simulink model "PV_solarpannel"  (R2019b)
settings: Solver=ode45  StartTime=0.0  StopTime=10.0  RelTol=1e-3  EnableMultiTasking=on
libraries: ee_lib x243, fl_lib x39, nesl_utility x11
(part 1 of 4)
settings Model: Creator=mm  LastModifiedBy=Rishabh
settings DataIOCC: LimitDataPoints=on  SaveFormat=Array  ReturnWorkspaceOutputs=off
settings OptimizationCC: LifeSpan=inf
settings DebuggingCC: SolverPrmCheckMsg=warning  SFUnexpectedBacktrackingDiag=warning  SFNoUnconditionalDefaultTransitionDiag=warning  SFExecutionAtInitializationDiag=none  ArithmeticOperatorsInVariantConditions=warning
settings HardwareCC: ProdBitPerPointer=32  ProdBitPerSizeT=32  ProdBitPerPtrDiffT=32  ProdLargestAtomicFloat=None  ProdIntDivRoundTo=Undefined  ProdEndianess=Unspecified  ProdWordSize=32  ProdHWDeviceType=32-bit Generic
settings ModelReferenceCC: PropagateSignalLabelsOutOfModel=off
settings SFSimCC: SimUseLocalCustomCode=off  CustomCodeUndefinedFunction=UseInterfaceOnly
settings RTWCC: RTWUseLocalCustomCode=off
settings CodeAppCC: StateflowObjectComments=on
settings GRTTargetCC: TargetLangStandard=C89/C90 (ANSI)  GeneratePreprocessorConditionals=Disable all
settings ConfigComp: CovMetricSettings=dw  CovHtmlReporting=on  CovSaveCumulativeToWorkspaceVar=on  CovSaveSingleToWorkspaceVar=on  CovExternalEMLEnable=off  CovSFcnEnable=off
settings SimscapeCC: SimscapeNormalizeSystem=off

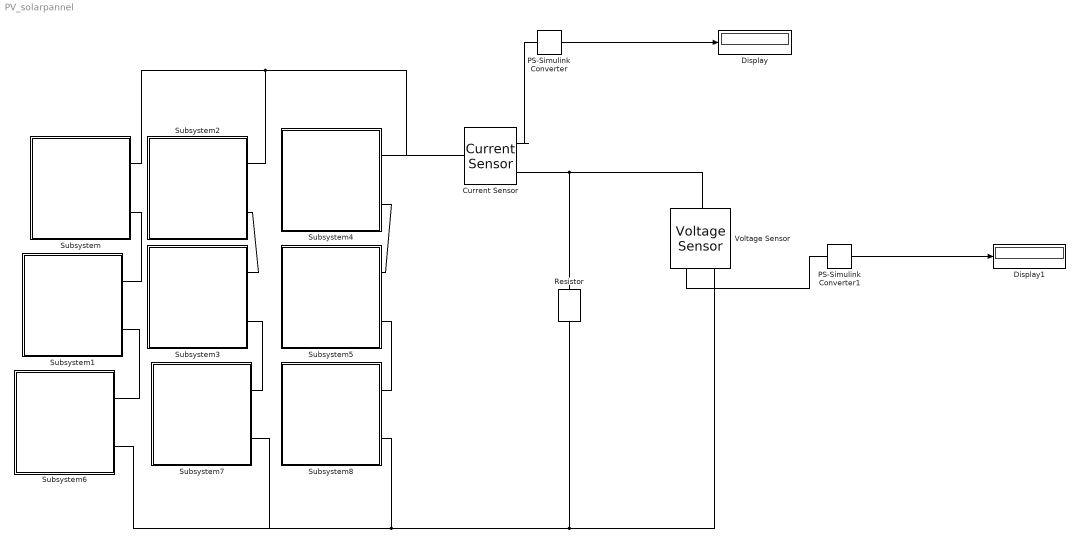
== system PV_solarpannel ==
  Current Sensor : fl_lib/Electrical/Electrical Sensors/Current Sensor
  Display : Display
  Display1 : Display
  PS-Simulink Converter : nesl_utility/PS-Simulink Converter  PhysicalDomain=network_engine_domain  SubClassName=ps_output  LeftPortType=input  RightPortType=output  PseudoPeriodic=off  Frequencies=[]  Unit=1  AffineConversion=off
  PS-Simulink Converter1 : nesl_utility/PS-Simulink Converter  PhysicalDomain=network_engine_domain  SubClassName=ps_output  LeftPortType=input  RightPortType=output  PseudoPeriodic=off  Frequencies=[]  Unit=1  AffineConversion=off
  Resistor : fl_lib/Electrical/Electrical Elements/Resistor  R=1 Ohm  i_specify=off  i_priority=High  i=0 A  i_nominal_specify=off  i_nominal_unit=A  i_nominal_value=1  v_specify=off  v_priority=High  v=0 V  v_nominal_specify=off  v_nominal_unit=V  v_nominal_value=1
  Subsystem : Subsystem
  Subsystem1 : Subsystem
  Subsystem2 : Subsystem
  Subsystem3 : Subsystem
  Subsystem4 : Subsystem
  Subsystem5 : Subsystem
  Subsystem6 : Subsystem
  Subsystem7 : Subsystem
  Subsystem8 : Subsystem
  Voltage Sensor : fl_lib/Electrical/Electrical Sensors/Voltage Sensor
  wires:
  PS-Simulink Converter/1 -> Display/1
  PS-Simulink Converter1/1 -> Display1/1
  connections:
  Current Sensor/RConn2 -- Voltage Sensor/LConn1 -- Resistor/LConn1
  Current Sensor/RConn1 -- PS-Simulink Converter/LConn1
  Voltage Sensor/RConn1 -- PS-Simulink Converter1/LConn1
  Resistor/RConn1 -- Subsystem7/RConn2 -- Subsystem6/RConn2 -- Subsystem8/RConn2 -- Voltage Sensor/RConn2
  Subsystem1/RConn1 -- Subsystem/RConn2
  Subsystem3/RConn1 -- Subsystem2/RConn2
  Subsystem3/RConn2 -- Subsystem7/RConn1
  Subsystem1/RConn2 -- Subsystem6/RConn1
  Subsystem5/RConn2 -- Subsystem8/RConn1
  Subsystem4/RConn2 -- Subsystem5/RConn1
  Subsystem/RConn1 -- Subsystem4/RConn1 -- Current Sensor/LConn1 -- Subsystem2/RConn1

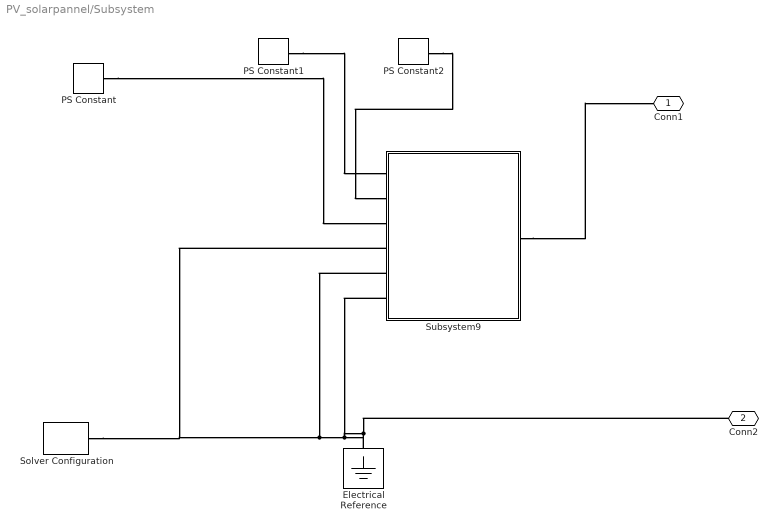
== system PV_solarpannel/Subsystem ==
  Electrical Reference : fl_lib/Electrical/Electrical Elements/Electrical Reference
  PS Constant : fl_lib/Physical Signals/Sources/PS Constant  constant=1000
  PS Constant1 : fl_lib/Physical Signals/Sources/PS Constant  constant=1000
  PS Constant2 : fl_lib/Physical Signals/Sources/PS Constant  constant=1000
  Solver Configuration : nesl_utility/Solver Configuration  PhysicalDomain=network_engine_domain  SubClassName=solver  LeftPortType=input  RightPortType=generic  Tones=[]  Harmonics=[]  SimulateNoise=off  Profile=off  UseLocalSampling=off  EnableSwitchedLinearOptims=on  FrequencyDomain=off  UseCCode=off  RelTol=0.001  AbsTol=1e-06  MinStep=1e-09  ToWorkspace=off  RevertToSquareIcSolve=off  NumHomotopyIterations=100  PhasorMode=off  PhasorModeNumHarmonics=1  DoDC=off  ResidualTolerance=1e-09  UseLocalSolver=off  LocalSolverChoice=NE_BACKWARD_EULER_ADVANCER  LocalSolverSampleTime=0.001  DoFixedCost=off  MaxNonlinIter=3  MaxModeIter=2  LinearAlgebra=Sparse  EquationFormulation=NE_TIME_EF  DelaysMemoryBudget=1024  AutomaticFiltering=on  FilteringTimeConstant=0.001  PartitionStorageMethod=AS_NEEDED  PartitionMemoryBudget=1024  PartitionMethod=FAST
  Subsystem9 : Subsystem
  Conn1 : PMIOPort  Side=Right
  Conn2 : PMIOPort  Port=2  Side=Right
  connections:
  Electrical Reference/LConn1 -- Subsystem9/LConn6 -- Subsystem9/LConn5 -- Subsystem9/LConn4 -- Solver Configuration/RConn1 -- Conn2/RConn1
  PS Constant1/RConn1 -- Subsystem9/LConn1
  PS Constant/RConn1 -- Subsystem9/LConn3
  PS Constant2/RConn1 -- Subsystem9/LConn2
  Subsystem9/RConn1 -- Conn1/RConn1

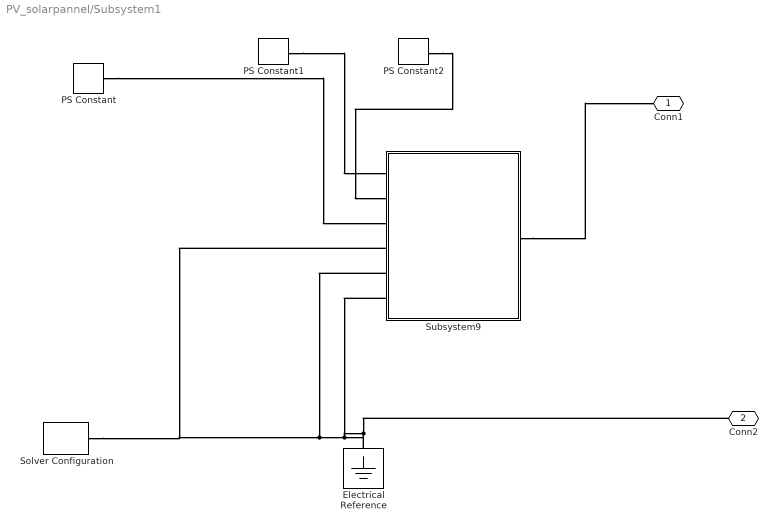
== system PV_solarpannel/Subsystem1 ==
  Electrical Reference : fl_lib/Electrical/Electrical Elements/Electrical Reference
  PS Constant : fl_lib/Physical Signals/Sources/PS Constant  constant=1000
  PS Constant1 : fl_lib/Physical Signals/Sources/PS Constant  constant=1000
  PS Constant2 : fl_lib/Physical Signals/Sources/PS Constant  constant=1000
  Solver Configuration : nesl_utility/Solver Configuration  PhysicalDomain=network_engine_domain  SubClassName=solver  LeftPortType=input  RightPortType=generic  Tones=[]  Harmonics=[]  SimulateNoise=off  Profile=off  UseLocalSampling=off  EnableSwitchedLinearOptims=on  FrequencyDomain=off  UseCCode=off  RelTol=0.001  AbsTol=1e-06  MinStep=1e-09  ToWorkspace=off  RevertToSquareIcSolve=off  NumHomotopyIterations=100  PhasorMode=off  PhasorModeNumHarmonics=1  DoDC=off  ResidualTolerance=1e-09  UseLocalSolver=off  LocalSolverChoice=NE_BACKWARD_EULER_ADVANCER  LocalSolverSampleTime=0.001  DoFixedCost=off  MaxNonlinIter=3  MaxModeIter=2  LinearAlgebra=Sparse  EquationFormulation=NE_TIME_EF  DelaysMemoryBudget=1024  AutomaticFiltering=on  FilteringTimeConstant=0.001  PartitionStorageMethod=AS_NEEDED  PartitionMemoryBudget=1024  PartitionMethod=FAST
  Subsystem9 : Subsystem
  Conn1 : PMIOPort  Side=Right
  Conn2 : PMIOPort  Port=2  Side=Right
  connections:
  Electrical Reference/LConn1 -- Subsystem9/LConn6 -- Subsystem9/LConn5 -- Subsystem9/LConn4 -- Solver Configuration/RConn1 -- Conn2/RConn1
  PS Constant1/RConn1 -- Subsystem9/LConn1
  PS Constant/RConn1 -- Subsystem9/LConn3
  PS Constant2/RConn1 -- Subsystem9/LConn2
  Subsystem9/RConn1 -- Conn1/RConn1

== system PV_solarpannel/Subsystem2 ==
  Electrical Reference : fl_lib/Electrical/Electrical Elements/Electrical Reference
  PS Constant : fl_lib/Physical Signals/Sources/PS Constant  constant=1000
  PS Constant1 : fl_lib/Physical Signals/Sources/PS Constant  constant=1000
  PS Constant2 : fl_lib/Physical Signals/Sources/PS Constant  constant=1000
  Solver Configuration : nesl_utility/Solver Configuration  PhysicalDomain=network_engine_domain  SubClassName=solver  LeftPortType=input  RightPortType=generic  Tones=[]  Harmonics=[]  SimulateNoise=off  Profile=off  UseLocalSampling=off  EnableSwitchedLinearOptims=on  FrequencyDomain=off  UseCCode=off  RelTol=0.001  AbsTol=1e-06  MinStep=1e-09  ToWorkspace=off  RevertToSquareIcSolve=off  NumHomotopyIterations=100  PhasorMode=off  PhasorModeNumHarmonics=1  DoDC=off  ResidualTolerance=1e-09  UseLocalSolver=off  LocalSolverChoice=NE_BACKWARD_EULER_ADVANCER  LocalSolverSampleTime=0.001  DoFixedCost=off  MaxNonlinIter=3  MaxModeIter=2  LinearAlgebra=Sparse  EquationFormulation=NE_TIME_EF  DelaysMemoryBudget=1024  AutomaticFiltering=on  FilteringTimeConstant=0.001  PartitionStorageMethod=AS_NEEDED  PartitionMemoryBudget=1024  PartitionMethod=FAST
  Subsystem9 : Subsystem
  Conn1 : PMIOPort  Side=Right
  Conn2 : PMIOPort  Port=2  Side=Right
  connections:
  Electrical Reference/LConn1 -- Subsystem9/LConn6 -- Subsystem9/LConn5 -- Subsystem9/LConn4 -- Solver Configuration/RConn1 -- Conn2/RConn1
  PS Constant1/RConn1 -- Subsystem9/LConn1
  PS Constant/RConn1 -- Subsystem9/LConn3
  PS Constant2/RConn1 -- Subsystem9/LConn2
  Subsystem9/RConn1 -- Conn1/RConn1

== system PV_solarpannel/Subsystem3 ==
  Electrical Reference : fl_lib/Electrical/Electrical Elements/Electrical Reference
  PS Constant : fl_lib/Physical Signals/Sources/PS Constant  constant=1000
  PS Constant1 : fl_lib/Physical Signals/Sources/PS Constant  constant=1000
  PS Constant2 : fl_lib/Physical Signals/Sources/PS Constant  constant=1000
  Solver Configuration : nesl_utility/Solver Configuration  PhysicalDomain=network_engine_domain  SubClassName=solver  LeftPortType=input  RightPortType=generic  Tones=[]  Harmonics=[]  SimulateNoise=off  Profile=off  UseLocalSampling=off  EnableSwitchedLinearOptims=on  FrequencyDomain=off  UseCCode=off  RelTol=0.001  AbsTol=1e-06  MinStep=1e-09  ToWorkspace=off  RevertToSquareIcSolve=off  NumHomotopyIterations=100  PhasorMode=off  PhasorModeNumHarmonics=1  DoDC=off  ResidualTolerance=1e-09  UseLocalSolver=off  LocalSolverChoice=NE_BACKWARD_EULER_ADVANCER  LocalSolverSampleTime=0.001  DoFixedCost=off  MaxNonlinIter=3  MaxModeIter=2  LinearAlgebra=Sparse  EquationFormulation=NE_TIME_EF  DelaysMemoryBudget=1024  AutomaticFiltering=on  FilteringTimeConstant=0.001  PartitionStorageMethod=AS_NEEDED  PartitionMemoryBudget=1024  PartitionMethod=FAST
  Subsystem9 : Subsystem
  Conn1 : PMIOPort  Side=Right
  Conn2 : PMIOPort  Port=2  Side=Right
  connections:
  Electrical Reference/LConn1 -- Subsystem9/LConn6 -- Subsystem9/LConn5 -- Subsystem9/LConn4 -- Solver Configuration/RConn1 -- Conn2/RConn1
  PS Constant1/RConn1 -- Subsystem9/LConn1
  PS Constant/RConn1 -- Subsystem9/LConn3
  PS Constant2/RConn1 -- Subsystem9/LConn2
  Subsystem9/RConn1 -- Conn1/RConn1

== system PV_solarpannel/Subsystem4 ==
  Electrical Reference : fl_lib/Electrical/Electrical Elements/Electrical Reference
  PS Constant : fl_lib/Physical Signals/Sources/PS Constant  constant=1000
  PS Constant1 : fl_lib/Physical Signals/Sources/PS Constant  constant=1000
  PS Constant2 : fl_lib/Physical Signals/Sources/PS Constant  constant=1000
  Solver Configuration : nesl_utility/Solver Configuration  PhysicalDomain=network_engine_domain  SubClassName=solver  LeftPortType=input  RightPortType=generic  Tones=[]  Harmonics=[]  SimulateNoise=off  Profile=off  UseLocalSampling=off  EnableSwitchedLinearOptims=on  FrequencyDomain=off  UseCCode=off  RelTol=0.001  AbsTol=1e-06  MinStep=1e-09  ToWorkspace=off  RevertToSquareIcSolve=off  NumHomotopyIterations=100  PhasorMode=off  PhasorModeNumHarmonics=1  DoDC=off  ResidualTolerance=1e-09  UseLocalSolver=off  LocalSolverChoice=NE_BACKWARD_EULER_ADVANCER  LocalSolverSampleTime=0.001  DoFixedCost=off  MaxNonlinIter=3  MaxModeIter=2  LinearAlgebra=Sparse  EquationFormulation=NE_TIME_EF  DelaysMemoryBudget=1024  AutomaticFiltering=on  FilteringTimeConstant=0.001  PartitionStorageMethod=AS_NEEDED  PartitionMemoryBudget=1024  PartitionMethod=FAST
  Subsystem9 : Subsystem
  Conn1 : PMIOPort  Side=Right
  Conn2 : PMIOPort  Port=2  Side=Right
  connections:
  Electrical Reference/LConn1 -- Subsystem9/LConn6 -- Subsystem9/LConn5 -- Subsystem9/LConn4 -- Solver Configuration/RConn1 -- Conn2/RConn1
  PS Constant1/RConn1 -- Subsystem9/LConn1
  PS Constant/RConn1 -- Subsystem9/LConn3
  PS Constant2/RConn1 -- Subsystem9/LConn2
  Subsystem9/RConn1 -- Conn1/RConn1

== system PV_solarpannel/Subsystem5 ==
  Electrical Reference : fl_lib/Electrical/Electrical Elements/Electrical Reference
  PS Constant : fl_lib/Physical Signals/Sources/PS Constant  constant=1000
  PS Constant1 : fl_lib/Physical Signals/Sources/PS Constant  constant=1000
  PS Constant2 : fl_lib/Physical Signals/Sources/PS Constant  constant=1000
  Solver Configuration : nesl_utility/Solver Configuration  PhysicalDomain=network_engine_domain  SubClassName=solver  LeftPortType=input  RightPortType=generic  Tones=[]  Harmonics=[]  SimulateNoise=off  Profile=off  UseLocalSampling=off  EnableSwitchedLinearOptims=on  FrequencyDomain=off  UseCCode=off  RelTol=0.001  AbsTol=1e-06  MinStep=1e-09  ToWorkspace=off  RevertToSquareIcSolve=off  NumHomotopyIterations=100  PhasorMode=off  PhasorModeNumHarmonics=1  DoDC=off  ResidualTolerance=1e-09  UseLocalSolver=off  LocalSolverChoice=NE_BACKWARD_EULER_ADVANCER  LocalSolverSampleTime=0.001  DoFixedCost=off  MaxNonlinIter=3  MaxModeIter=2  LinearAlgebra=Sparse  EquationFormulation=NE_TIME_EF  DelaysMemoryBudget=1024  AutomaticFiltering=on  FilteringTimeConstant=0.001  PartitionStorageMethod=AS_NEEDED  PartitionMemoryBudget=1024  PartitionMethod=FAST
  Subsystem9 : Subsystem
  Conn1 : PMIOPort  Side=Right
  Conn2 : PMIOPort  Port=2  Side=Right
  connections:
  Electrical Reference/LConn1 -- Subsystem9/LConn6 -- Subsystem9/LConn5 -- Subsystem9/LConn4 -- Solver Configuration/RConn1 -- Conn2/RConn1
  PS Constant1/RConn1 -- Subsystem9/LConn1
  PS Constant/RConn1 -- Subsystem9/LConn3
  PS Constant2/RConn1 -- Subsystem9/LConn2
  Subsystem9/RConn1 -- Conn1/RConn1

== system PV_solarpannel/Subsystem6 ==
  Electrical Reference : fl_lib/Electrical/Electrical Elements/Electrical Reference
  PS Constant : fl_lib/Physical Signals/Sources/PS Constant  constant=1000
  PS Constant1 : fl_lib/Physical Signals/Sources/PS Constant  constant=1000
  PS Constant2 : fl_lib/Physical Signals/Sources/PS Constant  constant=1000
  Solver Configuration : nesl_utility/Solver Configuration  PhysicalDomain=network_engine_domain  SubClassName=solver  LeftPortType=input  RightPortType=generic  Tones=[]  Harmonics=[]  SimulateNoise=off  Profile=off  UseLocalSampling=off  EnableSwitchedLinearOptims=on  FrequencyDomain=off  UseCCode=off  RelTol=0.001  AbsTol=1e-06  MinStep=1e-09  ToWorkspace=off  RevertToSquareIcSolve=off  NumHomotopyIterations=100  PhasorMode=off  PhasorModeNumHarmonics=1  DoDC=off  ResidualTolerance=1e-09  UseLocalSolver=off  LocalSolverChoice=NE_BACKWARD_EULER_ADVANCER  LocalSolverSampleTime=0.001  DoFixedCost=off  MaxNonlinIter=3  MaxModeIter=2  LinearAlgebra=Sparse  EquationFormulation=NE_TIME_EF  DelaysMemoryBudget=1024  AutomaticFiltering=on  FilteringTimeConstant=0.001  PartitionStorageMethod=AS_NEEDED  PartitionMemoryBudget=1024  PartitionMethod=FAST
  Subsystem9 : Subsystem
  Conn1 : PMIOPort  Side=Right
  Conn2 : PMIOPort  Port=2  Side=Right
  connections:
  Electrical Reference/LConn1 -- Subsystem9/LConn6 -- Subsystem9/LConn5 -- Subsystem9/LConn4 -- Solver Configuration/RConn1 -- Conn2/RConn1
  PS Constant1/RConn1 -- Subsystem9/LConn1
  PS Constant/RConn1 -- Subsystem9/LConn3
  PS Constant2/RConn1 -- Subsystem9/LConn2
  Subsystem9/RConn1 -- Conn1/RConn1

== system PV_solarpannel/Subsystem7 ==
  Electrical Reference : fl_lib/Electrical/Electrical Elements/Electrical Reference
  PS Constant : fl_lib/Physical Signals/Sources/PS Constant  constant=1000
  PS Constant1 : fl_lib/Physical Signals/Sources/PS Constant  constant=1000
  PS Constant2 : fl_lib/Physical Signals/Sources/PS Constant  constant=1000
  Solver Configuration : nesl_utility/Solver Configuration  PhysicalDomain=network_engine_domain  SubClassName=solver  LeftPortType=input  RightPortType=generic  Tones=[]  Harmonics=[]  SimulateNoise=off  Profile=off  UseLocalSampling=off  EnableSwitchedLinearOptims=on  FrequencyDomain=off  UseCCode=off  RelTol=0.001  AbsTol=1e-06  MinStep=1e-09  ToWorkspace=off  RevertToSquareIcSolve=off  NumHomotopyIterations=100  PhasorMode=off  PhasorModeNumHarmonics=1  DoDC=off  ResidualTolerance=1e-09  UseLocalSolver=off  LocalSolverChoice=NE_BACKWARD_EULER_ADVANCER  LocalSolverSampleTime=0.001  DoFixedCost=off  MaxNonlinIter=3  MaxModeIter=2  LinearAlgebra=Sparse  EquationFormulation=NE_TIME_EF  DelaysMemoryBudget=1024  AutomaticFiltering=on  FilteringTimeConstant=0.001  PartitionStorageMethod=AS_NEEDED  PartitionMemoryBudget=1024  PartitionMethod=FAST
  Subsystem9 : Subsystem
  Conn1 : PMIOPort  Side=Right
  Conn2 : PMIOPort  Port=2  Side=Right
  connections:
  Electrical Reference/LConn1 -- Subsystem9/LConn6 -- Subsystem9/LConn5 -- Subsystem9/LConn4 -- Solver Configuration/RConn1 -- Conn2/RConn1
  PS Constant1/RConn1 -- Subsystem9/LConn1
  PS Constant/RConn1 -- Subsystem9/LConn3
  PS Constant2/RConn1 -- Subsystem9/LConn2
  Subsystem9/RConn1 -- Conn1/RConn1

== system PV_solarpannel/Subsystem8 ==
  Electrical Reference : fl_lib/Electrical/Electrical Elements/Electrical Reference
  PS Constant : fl_lib/Physical Signals/Sources/PS Constant  constant=1000
  PS Constant1 : fl_lib/Physical Signals/Sources/PS Constant  constant=1000
  PS Constant2 : fl_lib/Physical Signals/Sources/PS Constant  constant=1000
  Solver Configuration : nesl_utility/Solver Configuration  PhysicalDomain=network_engine_domain  SubClassName=solver  LeftPortType=input  RightPortType=generic  Tones=[]  Harmonics=[]  SimulateNoise=off  Profile=off  UseLocalSampling=off  EnableSwitchedLinearOptims=on  FrequencyDomain=off  UseCCode=off  RelTol=0.001  AbsTol=1e-06  MinStep=1e-09  ToWorkspace=off  RevertToSquareIcSolve=off  NumHomotopyIterations=100  PhasorMode=off  PhasorModeNumHarmonics=1  DoDC=off  ResidualTolerance=1e-09  UseLocalSolver=off  LocalSolverChoice=NE_BACKWARD_EULER_ADVANCER  LocalSolverSampleTime=0.001  DoFixedCost=off  MaxNonlinIter=3  MaxModeIter=2  LinearAlgebra=Sparse  EquationFormulation=NE_TIME_EF  DelaysMemoryBudget=1024  AutomaticFiltering=on  FilteringTimeConstant=0.001  PartitionStorageMethod=AS_NEEDED  PartitionMemoryBudget=1024  PartitionMethod=FAST
  Subsystem9 : Subsystem
  Conn1 : PMIOPort  Side=Right
  Conn2 : PMIOPort  Port=2  Side=Right
  connections:
  Electrical Reference/LConn1 -- Subsystem9/LConn6 -- Subsystem9/LConn5 -- Subsystem9/LConn4 -- Solver Configuration/RConn1 -- Conn2/RConn1
  PS Constant1/RConn1 -- Subsystem9/LConn1
  PS Constant/RConn1 -- Subsystem9/LConn3
  PS Constant2/RConn1 -- Subsystem9/LConn2
  Subsystem9/RConn1 -- Conn1/RConn1

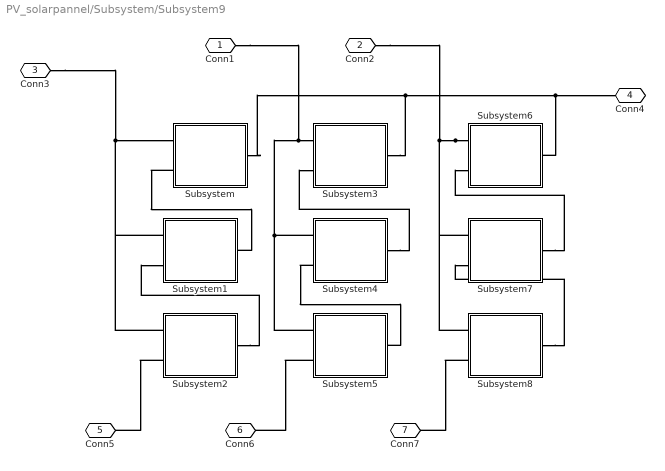
== system PV_solarpannel/Subsystem/Subsystem9 ==
  Subsystem : Subsystem
  Subsystem1 : Subsystem
  Subsystem2 : Subsystem
  Subsystem3 : Subsystem
  Subsystem4 : Subsystem
  Subsystem5 : Subsystem
  Subsystem6 : Subsystem
  Subsystem7 : Subsystem
  Subsystem8 : Subsystem
  Conn1 : PMIOPort  Side=Left
  Conn2 : PMIOPort  Port=2  Side=Left
  Conn3 : PMIOPort  Port=3  Side=Left
  Conn4 : PMIOPort  Port=4  Side=Right
  Conn5 : PMIOPort  Port=5  Side=Left
  Conn6 : PMIOPort  Port=6  Side=Left
  Conn7 : PMIOPort  Port=7  Side=Left
  connections:
  Subsystem3/RConn1 -- Subsystem/RConn1 -- Conn4/RConn1 -- Subsystem6/RConn1
  Subsystem6/LConn1 -- Conn2/RConn1 -- Subsystem8/LConn1 -- Subsystem7/LConn1
  Subsystem8/RConn1 -- Subsystem7/LConn2
  Subsystem4/LConn1 -- Conn1/RConn1 -- Subsystem3/LConn1 -- Subsystem5/LConn1
  Subsystem2/LConn2 -- Conn5/RConn1
  Subsystem/LConn2 -- Subsystem1/RConn1
  Subsystem7/RConn1 -- Subsystem6/LConn2
  Subsystem2/LConn1 -- Subsystem1/LConn1 -- Conn3/RConn1 -- Subsystem/LConn1
  Subsystem2/RConn1 -- Subsystem1/LConn2
  Subsystem4/RConn1 -- Subsystem3/LConn2
  Subsystem4/LConn2 -- Subsystem5/RConn1
  Subsystem8/LConn2 -- Conn7/RConn1
  Subsystem5/LConn2 -- Conn6/RConn1

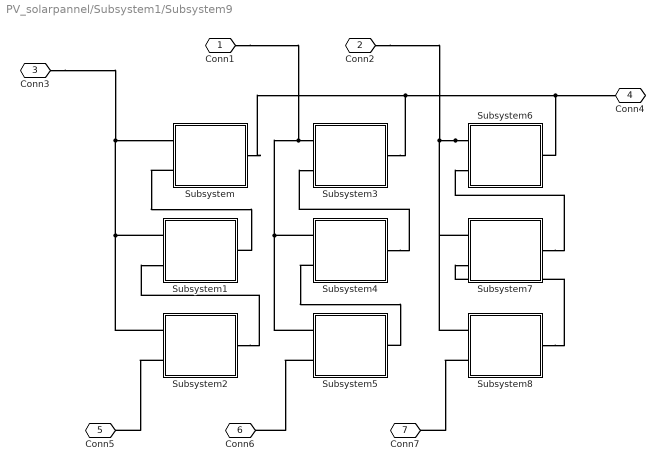
== system PV_solarpannel/Subsystem1/Subsystem9 ==
  Subsystem : Subsystem
  Subsystem1 : Subsystem
  Subsystem2 : Subsystem
  Subsystem3 : Subsystem
  Subsystem4 : Subsystem
  Subsystem5 : Subsystem
  Subsystem6 : Subsystem
  Subsystem7 : Subsystem
  Subsystem8 : Subsystem
  Conn1 : PMIOPort  Side=Left
  Conn2 : PMIOPort  Port=2  Side=Left
  Conn3 : PMIOPort  Port=3  Side=Left
  Conn4 : PMIOPort  Port=4  Side=Right
  Conn5 : PMIOPort  Port=5  Side=Left
  Conn6 : PMIOPort  Port=6  Side=Left
  Conn7 : PMIOPort  Port=7  Side=Left
  connections:
  Subsystem3/RConn1 -- Subsystem/RConn1 -- Conn4/RConn1 -- Subsystem6/RConn1
  Subsystem6/LConn1 -- Conn2/RConn1 -- Subsystem8/LConn1 -- Subsystem7/LConn1
  Subsystem8/RConn1 -- Subsystem7/LConn2
  Subsystem4/LConn1 -- Conn1/RConn1 -- Subsystem3/LConn1 -- Subsystem5/LConn1
  Subsystem2/LConn2 -- Conn5/RConn1
  Subsystem/LConn2 -- Subsystem1/RConn1
  Subsystem7/RConn1 -- Subsystem6/LConn2
  Subsystem2/LConn1 -- Subsystem1/LConn1 -- Conn3/RConn1 -- Subsystem/LConn1
  Subsystem2/RConn1 -- Subsystem1/LConn2
  Subsystem4/RConn1 -- Subsystem3/LConn2
  Subsystem4/LConn2 -- Subsystem5/RConn1
  Subsystem8/LConn2 -- Conn7/RConn1
  Subsystem5/LConn2 -- Conn6/RConn1

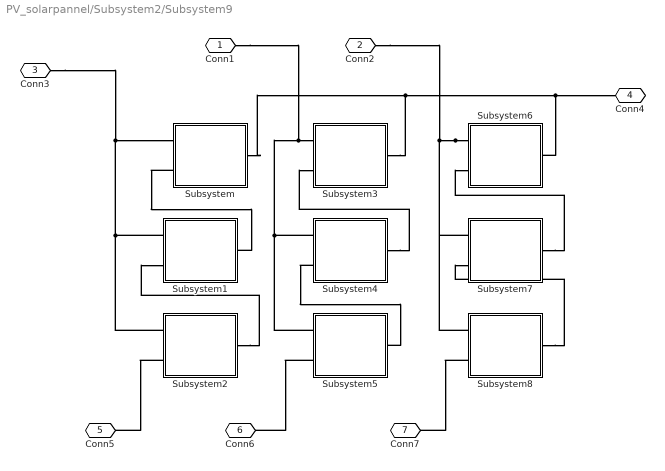
== system PV_solarpannel/Subsystem2/Subsystem9 ==
  Subsystem : Subsystem
  Subsystem1 : Subsystem
  Subsystem2 : Subsystem
  Subsystem3 : Subsystem
  Subsystem4 : Subsystem
  Subsystem5 : Subsystem
  Subsystem6 : Subsystem
  Subsystem7 : Subsystem
  Subsystem8 : Subsystem
  Conn1 : PMIOPort  Side=Left
  Conn2 : PMIOPort  Port=2  Side=Left
  Conn3 : PMIOPort  Port=3  Side=Left
  Conn4 : PMIOPort  Port=4  Side=Right
  Conn5 : PMIOPort  Port=5  Side=Left
  Conn6 : PMIOPort  Port=6  Side=Left
  Conn7 : PMIOPort  Port=7  Side=Left
  connections:
  Subsystem3/RConn1 -- Subsystem/RConn1 -- Conn4/RConn1 -- Subsystem6/RConn1
  Subsystem6/LConn1 -- Conn2/RConn1 -- Subsystem8/LConn1 -- Subsystem7/LConn1
  Subsystem8/RConn1 -- Subsystem7/LConn2
  Subsystem4/LConn1 -- Conn1/RConn1 -- Subsystem3/LConn1 -- Subsystem5/LConn1
  Subsystem2/LConn2 -- Conn5/RConn1
  Subsystem/LConn2 -- Subsystem1/RConn1
  Subsystem7/RConn1 -- Subsystem6/LConn2
  Subsystem2/LConn1 -- Subsystem1/LConn1 -- Conn3/RConn1 -- Subsystem/LConn1
  Subsystem2/RConn1 -- Subsystem1/LConn2
  Subsystem4/RConn1 -- Subsystem3/LConn2
  Subsystem4/LConn2 -- Subsystem5/RConn1
  Subsystem8/LConn2 -- Conn7/RConn1
  Subsystem5/LConn2 -- Conn6/RConn1

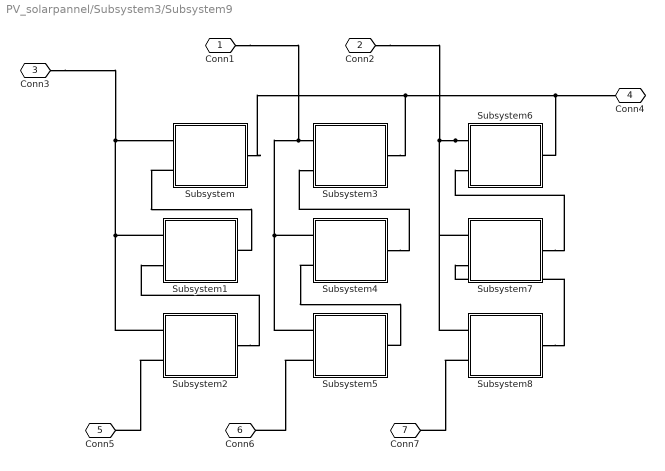
== system PV_solarpannel/Subsystem3/Subsystem9 ==
  Subsystem : Subsystem
  Subsystem1 : Subsystem
  Subsystem2 : Subsystem
  Subsystem3 : Subsystem
  Subsystem4 : Subsystem
  Subsystem5 : Subsystem
  Subsystem6 : Subsystem
  Subsystem7 : Subsystem
  Subsystem8 : Subsystem
  Conn1 : PMIOPort  Side=Left
  Conn2 : PMIOPort  Port=2  Side=Left
  Conn3 : PMIOPort  Port=3  Side=Left
  Conn4 : PMIOPort  Port=4  Side=Right
  Conn5 : PMIOPort  Port=5  Side=Left
  Conn6 : PMIOPort  Port=6  Side=Left
  Conn7 : PMIOPort  Port=7  Side=Left
  connections:
  Subsystem3/RConn1 -- Subsystem/RConn1 -- Conn4/RConn1 -- Subsystem6/RConn1
  Subsystem6/LConn1 -- Conn2/RConn1 -- Subsystem8/LConn1 -- Subsystem7/LConn1
  Subsystem8/RConn1 -- Subsystem7/LConn2
  Subsystem4/LConn1 -- Conn1/RConn1 -- Subsystem3/LConn1 -- Subsystem5/LConn1
  Subsystem2/LConn2 -- Conn5/RConn1
  Subsystem/LConn2 -- Subsystem1/RConn1
  Subsystem7/RConn1 -- Subsystem6/LConn2
  Subsystem2/LConn1 -- Subsystem1/LConn1 -- Conn3/RConn1 -- Subsystem/LConn1
  Subsystem2/RConn1 -- Subsystem1/LConn2
  Subsystem4/RConn1 -- Subsystem3/LConn2
  Subsystem4/LConn2 -- Subsystem5/RConn1
  Subsystem8/LConn2 -- Conn7/RConn1
  Subsystem5/LConn2 -- Conn6/RConn1

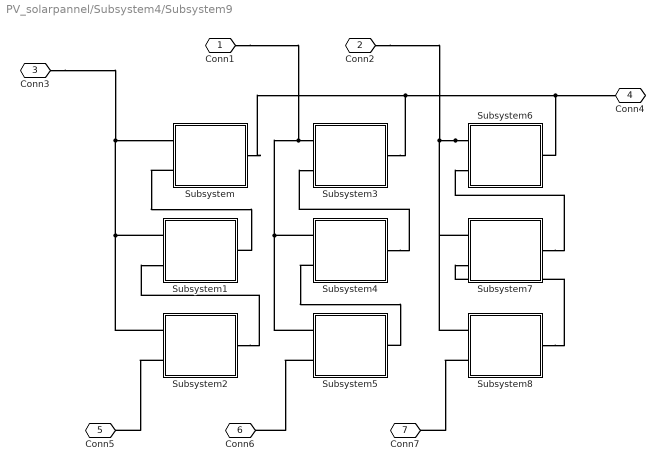
== system PV_solarpannel/Subsystem4/Subsystem9 ==
  Subsystem : Subsystem
  Subsystem1 : Subsystem
  Subsystem2 : Subsystem
  Subsystem3 : Subsystem
  Subsystem4 : Subsystem
  Subsystem5 : Subsystem
  Subsystem6 : Subsystem
  Subsystem7 : Subsystem
  Subsystem8 : Subsystem
  Conn1 : PMIOPort  Side=Left
  Conn2 : PMIOPort  Port=2  Side=Left
  Conn3 : PMIOPort  Port=3  Side=Left
  Conn4 : PMIOPort  Port=4  Side=Right
  Conn5 : PMIOPort  Port=5  Side=Left
  Conn6 : PMIOPort  Port=6  Side=Left
  Conn7 : PMIOPort  Port=7  Side=Left
  connections:
  Subsystem3/RConn1 -- Subsystem/RConn1 -- Conn4/RConn1 -- Subsystem6/RConn1
  Subsystem6/LConn1 -- Conn2/RConn1 -- Subsystem8/LConn1 -- Subsystem7/LConn1
  Subsystem8/RConn1 -- Subsystem7/LConn2
  Subsystem4/LConn1 -- Conn1/RConn1 -- Subsystem3/LConn1 -- Subsystem5/LConn1
  Subsystem2/LConn2 -- Conn5/RConn1
  Subsystem/LConn2 -- Subsystem1/RConn1
  Subsystem7/RConn1 -- Subsystem6/LConn2
  Subsystem2/LConn1 -- Subsystem1/LConn1 -- Conn3/RConn1 -- Subsystem/LConn1
  Subsystem2/RConn1 -- Subsystem1/LConn2
  Subsystem4/RConn1 -- Subsystem3/LConn2
  Subsystem4/LConn2 -- Subsystem5/RConn1
  Subsystem8/LConn2 -- Conn7/RConn1
  Subsystem5/LConn2 -- Conn6/RConn1

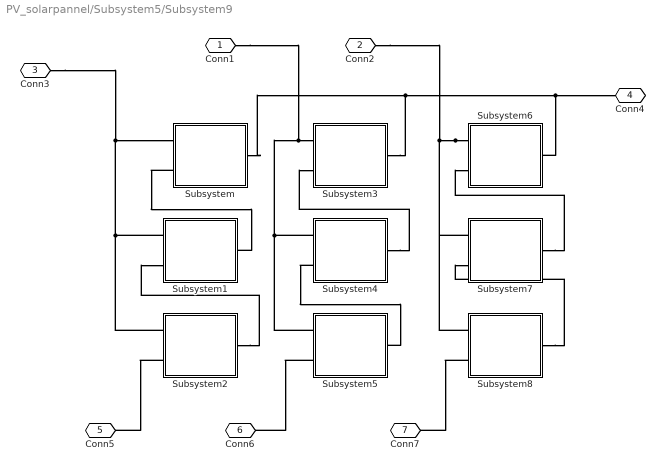
== system PV_solarpannel/Subsystem5/Subsystem9 ==
  Subsystem : Subsystem
  Subsystem1 : Subsystem
  Subsystem2 : Subsystem
  Subsystem3 : Subsystem
  Subsystem4 : Subsystem
  Subsystem5 : Subsystem
  Subsystem6 : Subsystem
  Subsystem7 : Subsystem
  Subsystem8 : Subsystem
  Conn1 : PMIOPort  Side=Left
  Conn2 : PMIOPort  Port=2  Side=Left
  Conn3 : PMIOPort  Port=3  Side=Left
  Conn4 : PMIOPort  Port=4  Side=Right
  Conn5 : PMIOPort  Port=5  Side=Left
  Conn6 : PMIOPort  Port=6  Side=Left
  Conn7 : PMIOPort  Port=7  Side=Left
  connections:
  Subsystem3/RConn1 -- Subsystem/RConn1 -- Conn4/RConn1 -- Subsystem6/RConn1
  Subsystem6/LConn1 -- Conn2/RConn1 -- Subsystem8/LConn1 -- Subsystem7/LConn1
  Subsystem8/RConn1 -- Subsystem7/LConn2
  Subsystem4/LConn1 -- Conn1/RConn1 -- Subsystem3/LConn1 -- Subsystem5/LConn1
  Subsystem2/LConn2 -- Conn5/RConn1
  Subsystem/LConn2 -- Subsystem1/RConn1
  Subsystem7/RConn1 -- Subsystem6/LConn2
  Subsystem2/LConn1 -- Subsystem1/LConn1 -- Conn3/RConn1 -- Subsystem/LConn1
  Subsystem2/RConn1 -- Subsystem1/LConn2
  Subsystem4/RConn1 -- Subsystem3/LConn2
  Subsystem4/LConn2 -- Subsystem5/RConn1
  Subsystem8/LConn2 -- Conn7/RConn1
  Subsystem5/LConn2 -- Conn6/RConn1

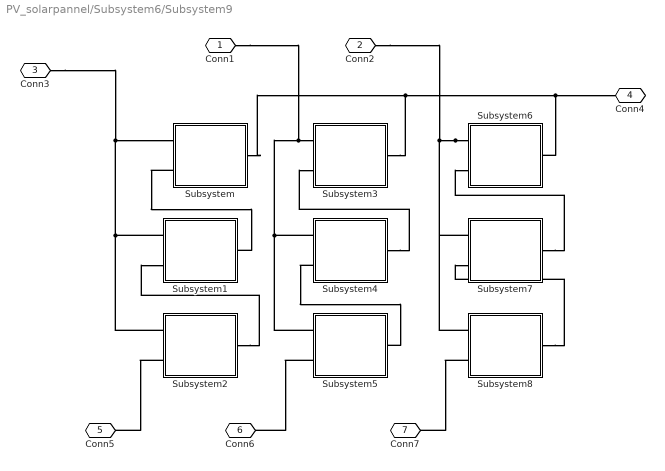
== system PV_solarpannel/Subsystem6/Subsystem9 ==
  Subsystem : Subsystem
  Subsystem1 : Subsystem
  Subsystem2 : Subsystem
  Subsystem3 : Subsystem
  Subsystem4 : Subsystem
  Subsystem5 : Subsystem
  Subsystem6 : Subsystem
  Subsystem7 : Subsystem
  Subsystem8 : Subsystem
  Conn1 : PMIOPort  Side=Left
  Conn2 : PMIOPort  Port=2  Side=Left
  Conn3 : PMIOPort  Port=3  Side=Left
  Conn4 : PMIOPort  Port=4  Side=Right
  Conn5 : PMIOPort  Port=5  Side=Left
  Conn6 : PMIOPort  Port=6  Side=Left
  Conn7 : PMIOPort  Port=7  Side=Left
  connections:
  Subsystem3/RConn1 -- Subsystem/RConn1 -- Conn4/RConn1 -- Subsystem6/RConn1
  Subsystem6/LConn1 -- Conn2/RConn1 -- Subsystem8/LConn1 -- Subsystem7/LConn1
  Subsystem8/RConn1 -- Subsystem7/LConn2
  Subsystem4/LConn1 -- Conn1/RConn1 -- Subsystem3/LConn1 -- Subsystem5/LConn1
  Subsystem2/LConn2 -- Conn5/RConn1
  Subsystem/LConn2 -- Subsystem1/RConn1
  Subsystem7/RConn1 -- Subsystem6/LConn2
  Subsystem2/LConn1 -- Subsystem1/LConn1 -- Conn3/RConn1 -- Subsystem/LConn1
  Subsystem2/RConn1 -- Subsystem1/LConn2
  Subsystem4/RConn1 -- Subsystem3/LConn2
  Subsystem4/LConn2 -- Subsystem5/RConn1
  Subsystem8/LConn2 -- Conn7/RConn1
  Subsystem5/LConn2 -- Conn6/RConn1

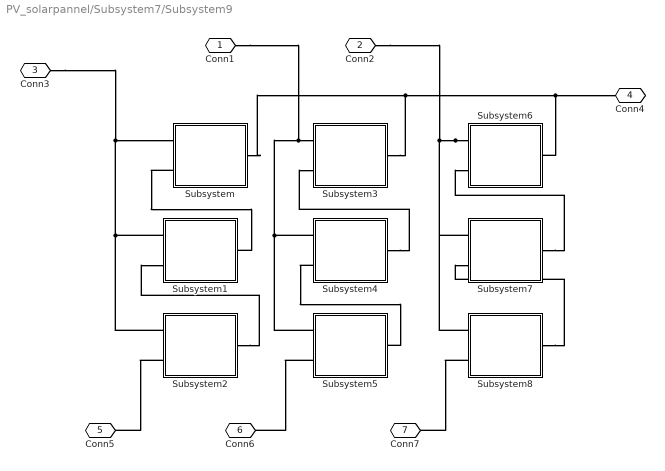
== system PV_solarpannel/Subsystem7/Subsystem9 ==
  Subsystem : Subsystem
  Subsystem1 : Subsystem
  Subsystem2 : Subsystem
  Subsystem3 : Subsystem
  Subsystem4 : Subsystem
  Subsystem5 : Subsystem
  Subsystem6 : Subsystem
  Subsystem7 : Subsystem
  Subsystem8 : Subsystem
  Conn1 : PMIOPort  Side=Left
  Conn2 : PMIOPort  Port=2  Side=Left
  Conn3 : PMIOPort  Port=3  Side=Left
  Conn4 : PMIOPort  Port=4  Side=Right
  Conn5 : PMIOPort  Port=5  Side=Left
  Conn6 : PMIOPort  Port=6  Side=Left
  Conn7 : PMIOPort  Port=7  Side=Left
  connections:
  Subsystem3/RConn1 -- Subsystem/RConn1 -- Conn4/RConn1 -- Subsystem6/RConn1
  Subsystem6/LConn1 -- Conn2/RConn1 -- Subsystem8/LConn1 -- Subsystem7/LConn1
  Subsystem8/RConn1 -- Subsystem7/LConn2
  Subsystem4/LConn1 -- Conn1/RConn1 -- Subsystem3/LConn1 -- Subsystem5/LConn1
  Subsystem2/LConn2 -- Conn5/RConn1
  Subsystem/LConn2 -- Subsystem1/RConn1
  Subsystem7/RConn1 -- Subsystem6/LConn2
  Subsystem2/LConn1 -- Subsystem1/LConn1 -- Conn3/RConn1 -- Subsystem/LConn1
  Subsystem2/RConn1 -- Subsystem1/LConn2
  Subsystem4/RConn1 -- Subsystem3/LConn2
  Subsystem4/LConn2 -- Subsystem5/RConn1
  Subsystem8/LConn2 -- Conn7/RConn1
  Subsystem5/LConn2 -- Conn6/RConn1

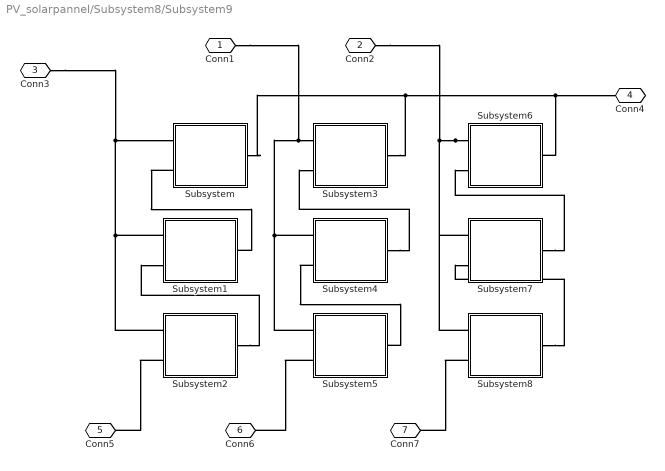
== system PV_solarpannel/Subsystem8/Subsystem9 ==
  Subsystem : Subsystem
  Subsystem1 : Subsystem
  Subsystem2 : Subsystem
  Subsystem3 : Subsystem
  Subsystem4 : Subsystem
  Subsystem5 : Subsystem
  Subsystem6 : Subsystem
  Subsystem7 : Subsystem
  Subsystem8 : Subsystem
  Conn1 : PMIOPort  Side=Left
  Conn2 : PMIOPort  Port=2  Side=Left
  Conn3 : PMIOPort  Port=3  Side=Left
  Conn4 : PMIOPort  Port=4  Side=Right
  Conn5 : PMIOPort  Port=5  Side=Left
  Conn6 : PMIOPort  Port=6  Side=Left
  Conn7 : PMIOPort  Port=7  Side=Left
  connections:
  Subsystem3/RConn1 -- Subsystem/RConn1 -- Conn4/RConn1 -- Subsystem6/RConn1
  Subsystem6/LConn1 -- Conn2/RConn1 -- Subsystem8/LConn1 -- Subsystem7/LConn1
  Subsystem8/RConn1 -- Subsystem7/LConn2
  Subsystem4/LConn1 -- Conn1/RConn1 -- Subsystem3/LConn1 -- Subsystem5/LConn1
  Subsystem2/LConn2 -- Conn5/RConn1
  Subsystem/LConn2 -- Subsystem1/RConn1
  Subsystem7/RConn1 -- Subsystem6/LConn2
  Subsystem2/LConn1 -- Subsystem1/LConn1 -- Conn3/RConn1 -- Subsystem/LConn1
  Subsystem2/RConn1 -- Subsystem1/LConn2
  Subsystem4/RConn1 -- Subsystem3/LConn2
  Subsystem4/LConn2 -- Subsystem5/RConn1
  Subsystem8/LConn2 -- Conn7/RConn1
  Subsystem5/LConn2 -- Conn6/RConn1

== system PV_solarpannel/Subsystem/Subsystem9/Subsystem ==
  Solar Cell : ee_lib/Sources/Solar Cell  prm=1  Isc=6 A  Voc=0.6 V  Is=1e-6 A  Is2=0 A  Iph=7.34 A  Ir0=1000 W/m^2  ec=1.5  N2=2  Rs=0 Ohm  Rp=Inf Ohm  N_series=1  TIPH1=0 1/K  EG=1.11 eV  TXIS1=3  TXIS2=3  TRS1=0  TRP1=0  Tmeas=25 C  TFIXED=25 C  thermal_mass=100 J/K  initial_temperature=25 degC
      settings: SourceProductName=Simscape Electrical  SourceProductBaseCode=PS
  Solar Cell1 : ee_lib/Sources/Solar Cell  prm=1  Isc=6 A  Voc=0.6 V  Is=1e-6 A  Is2=0 A  Iph=7.34 A  Ir0=1000 W/m^2  ec=1.5  N2=2  Rs=0 Ohm  Rp=Inf Ohm  N_series=1  TIPH1=0 1/K  EG=1.11 eV  TXIS1=3  TXIS2=3  TRS1=0  TRP1=0  Tmeas=25 C  TFIXED=25 C  thermal_mass=100 J/K  initial_temperature=25 degC
      settings: SourceProductName=Simscape Electrical  SourceProductBaseCode=PS
  Solar Cell2 : ee_lib/Sources/Solar Cell  prm=1  Isc=6 A  Voc=0.6 V  Is=1e-6 A  Is2=0 A  Iph=7.34 A  Ir0=1000 W/m^2  ec=1.5  N2=2  Rs=0 Ohm  Rp=Inf Ohm  N_series=1  TIPH1=0 1/K  EG=1.11 eV  TXIS1=3  TXIS2=3  TRS1=0  TRP1=0  Tmeas=25 C  TFIXED=25 C  thermal_mass=100 J/K  initial_temperature=25 degC
      settings: SourceProductName=Simscape Electrical  SourceProductBaseCode=PS
  Conn1 : PMIOPort  Side=Left
  Conn2 : PMIOPort  Port=2  Side=Right
  Conn3 : PMIOPort  Port=3  Side=Left
  connections:
  Solar Cell/LConn2 -- Conn2/RConn1
  Solar Cell/LConn1 -- Conn1/RConn1 -- Solar Cell2/LConn1 -- Solar Cell1/LConn1
  Solar Cell1/RConn1 -- Solar Cell2/LConn2
  Solar Cell/RConn1 -- Solar Cell1/LConn2
  Solar Cell2/RConn1 -- Conn3/RConn1

== system PV_solarpannel/Subsystem/Subsystem9/Subsystem1 ==
  Solar Cell : ee_lib/Sources/Solar Cell  prm=1  Isc=6 A  Voc=0.6 V  Is=1e-6 A  Is2=0 A  Iph=7.34 A  Ir0=1000 W/m^2  ec=1.5  N2=2  Rs=0 Ohm  Rp=Inf Ohm  N_series=1  TIPH1=0 1/K  EG=1.11 eV  TXIS1=3  TXIS2=3  TRS1=0  TRP1=0  Tmeas=25 C  TFIXED=25 C  thermal_mass=100 J/K  initial_temperature=25 degC
      settings: SourceProductName=Simscape Electrical  SourceProductBaseCode=PS
  Solar Cell1 : ee_lib/Sources/Solar Cell  prm=1  Isc=6 A  Voc=0.6 V  Is=1e-6 A  Is2=0 A  Iph=7.34 A  Ir0=1000 W/m^2  ec=1.5  N2=2  Rs=0 Ohm  Rp=Inf Ohm  N_series=1  TIPH1=0 1/K  EG=1.11 eV  TXIS1=3  TXIS2=3  TRS1=0  TRP1=0  Tmeas=25 C  TFIXED=25 C  thermal_mass=100 J/K  initial_temperature=25 degC
      settings: SourceProductName=Simscape Electrical  SourceProductBaseCode=PS
  Solar Cell2 : ee_lib/Sources/Solar Cell  prm=1  Isc=6 A  Voc=0.6 V  Is=1e-6 A  Is2=0 A  Iph=7.34 A  Ir0=1000 W/m^2  ec=1.5  N2=2  Rs=0 Ohm  Rp=Inf Ohm  N_series=1  TIPH1=0 1/K  EG=1.11 eV  TXIS1=3  TXIS2=3  TRS1=0  TRP1=0  Tmeas=25 C  TFIXED=25 C  thermal_mass=100 J/K  initial_temperature=25 degC
      settings: SourceProductName=Simscape Electrical  SourceProductBaseCode=PS
  Conn1 : PMIOPort  Side=Left
  Conn2 : PMIOPort  Port=2  Side=Right
  Conn3 : PMIOPort  Port=3  Side=Left
  connections:
  Solar Cell2/RConn1 -- Conn3/RConn1
  Solar Cell/RConn1 -- Solar Cell1/LConn2
  Solar Cell1/RConn1 -- Solar Cell2/LConn2
  Conn1/RConn1 -- Solar Cell/LConn1 -- Solar Cell1/LConn1 -- Solar Cell2/LConn1
  Solar Cell/LConn2 -- Conn2/RConn1

== system PV_solarpannel/Subsystem/Subsystem9/Subsystem2 ==
  Solar Cell : ee_lib/Sources/Solar Cell  prm=1  Isc=6 A  Voc=0.6 V  Is=1e-6 A  Is2=0 A  Iph=7.34 A  Ir0=1000 W/m^2  ec=1.5  N2=2  Rs=0 Ohm  Rp=Inf Ohm  N_series=1  TIPH1=0 1/K  EG=1.11 eV  TXIS1=3  TXIS2=3  TRS1=0  TRP1=0  Tmeas=25 C  TFIXED=25 C  thermal_mass=100 J/K  initial_temperature=25 degC
      settings: SourceProductName=Simscape Electrical  SourceProductBaseCode=PS
  Solar Cell1 : ee_lib/Sources/Solar Cell  prm=1  Isc=6 A  Voc=0.6 V  Is=1e-6 A  Is2=0 A  Iph=7.34 A  Ir0=1000 W/m^2  ec=1.5  N2=2  Rs=0 Ohm  Rp=Inf Ohm  N_series=1  TIPH1=0 1/K  EG=1.11 eV  TXIS1=3  TXIS2=3  TRS1=0  TRP1=0  Tmeas=25 C  TFIXED=25 C  thermal_mass=100 J/K  initial_temperature=25 degC
      settings: SourceProductName=Simscape Electrical  SourceProductBaseCode=PS
  Solar Cell2 : ee_lib/Sources/Solar Cell  prm=1  Isc=6 A  Voc=0.6 V  Is=1e-6 A  Is2=0 A  Iph=7.34 A  Ir0=1000 W/m^2  ec=1.5  N2=2  Rs=0 Ohm  Rp=Inf Ohm  N_series=1  TIPH1=0 1/K  EG=1.11 eV  TXIS1=3  TXIS2=3  TRS1=0  TRP1=0  Tmeas=25 C  TFIXED=25 C  thermal_mass=100 J/K  initial_temperature=25 degC
      settings: SourceProductName=Simscape Electrical  SourceProductBaseCode=PS
  Conn1 : PMIOPort  Side=Left
  Conn2 : PMIOPort  Port=2  Side=Right
  Conn3 : PMIOPort  Port=3  Side=Left
  connections:
  Solar Cell/LConn2 -- Conn2/RConn1
  Solar Cell2/LConn1 -- Solar Cell1/LConn1 -- Solar Cell/LConn1 -- Conn1/RConn1
  Solar Cell1/RConn1 -- Solar Cell2/LConn2
  Solar Cell/RConn1 -- Solar Cell1/LConn2
  Solar Cell2/RConn1 -- Conn3/RConn1

== system PV_solarpannel/Subsystem/Subsystem9/Subsystem3 ==
  Solar Cell : ee_lib/Sources/Solar Cell  prm=1  Isc=6 A  Voc=0.6 V  Is=1e-6 A  Is2=0 A  Iph=7.34 A  Ir0=1000 W/m^2  ec=1.5  N2=2  Rs=0 Ohm  Rp=Inf Ohm  N_series=1  TIPH1=0 1/K  EG=1.11 eV  TXIS1=3  TXIS2=3  TRS1=0  TRP1=0  Tmeas=25 C  TFIXED=25 C  thermal_mass=100 J/K  initial_temperature=25 degC
      settings: SourceProductName=Simscape Electrical  SourceProductBaseCode=PS
  Solar Cell1 : ee_lib/Sources/Solar Cell  prm=1  Isc=6 A  Voc=0.6 V  Is=1e-6 A  Is2=0 A  Iph=7.34 A  Ir0=1000 W/m^2  ec=1.5  N2=2  Rs=0 Ohm  Rp=Inf Ohm  N_series=1  TIPH1=0 1/K  EG=1.11 eV  TXIS1=3  TXIS2=3  TRS1=0  TRP1=0  Tmeas=25 C  TFIXED=25 C  thermal_mass=100 J/K  initial_temperature=25 degC
      settings: SourceProductName=Simscape Electrical  SourceProductBaseCode=PS
  Solar Cell2 : ee_lib/Sources/Solar Cell  prm=1  Isc=6 A  Voc=0.6 V  Is=1e-6 A  Is2=0 A  Iph=7.34 A  Ir0=1000 W/m^2  ec=1.5  N2=2  Rs=0 Ohm  Rp=Inf Ohm  N_series=1  TIPH1=0 1/K  EG=1.11 eV  TXIS1=3  TXIS2=3  TRS1=0  TRP1=0  Tmeas=25 C  TFIXED=25 C  thermal_mass=100 J/K  initial_temperature=25 degC
      settings: SourceProductName=Simscape Electrical  SourceProductBaseCode=PS
  Conn1 : PMIOPort  Side=Left
  Conn2 : PMIOPort  Port=2  Side=Right
  Conn3 : PMIOPort  Port=3  Side=Left
  connections:
  Solar Cell/LConn2 -- Conn2/RConn1
  Solar Cell/LConn1 -- Conn1/RConn1 -- Solar Cell2/LConn1 -- Solar Cell1/LConn1
  Solar Cell1/RConn1 -- Solar Cell2/LConn2
  Solar Cell/RConn1 -- Solar Cell1/LConn2
  Solar Cell2/RConn1 -- Conn3/RConn1

== system PV_solarpannel/Subsystem/Subsystem9/Subsystem4 ==
  Solar Cell : ee_lib/Sources/Solar Cell  prm=1  Isc=6 A  Voc=0.6 V  Is=1e-6 A  Is2=0 A  Iph=7.34 A  Ir0=1000 W/m^2  ec=1.5  N2=2  Rs=0 Ohm  Rp=Inf Ohm  N_series=1  TIPH1=0 1/K  EG=1.11 eV  TXIS1=3  TXIS2=3  TRS1=0  TRP1=0  Tmeas=25 C  TFIXED=25 C  thermal_mass=100 J/K  initial_temperature=25 degC
      settings: SourceProductName=Simscape Electrical  SourceProductBaseCode=PS
  Solar Cell1 : ee_lib/Sources/Solar Cell  prm=1  Isc=6 A  Voc=0.6 V  Is=1e-6 A  Is2=0 A  Iph=7.34 A  Ir0=1000 W/m^2  ec=1.5  N2=2  Rs=0 Ohm  Rp=Inf Ohm  N_series=1  TIPH1=0 1/K  EG=1.11 eV  TXIS1=3  TXIS2=3  TRS1=0  TRP1=0  Tmeas=25 C  TFIXED=25 C  thermal_mass=100 J/K  initial_temperature=25 degC
      settings: SourceProductName=Simscape Electrical  SourceProductBaseCode=PS
  Solar Cell2 : ee_lib/Sources/Solar Cell  prm=1  Isc=6 A  Voc=0.6 V  Is=1e-6 A  Is2=0 A  Iph=7.34 A  Ir0=1000 W/m^2  ec=1.5  N2=2  Rs=0 Ohm  Rp=Inf Ohm  N_series=1  TIPH1=0 1/K  EG=1.11 eV  TXIS1=3  TXIS2=3  TRS1=0  TRP1=0  Tmeas=25 C  TFIXED=25 C  thermal_mass=100 J/K  initial_temperature=25 degC
      settings: SourceProductName=Simscape Electrical  SourceProductBaseCode=PS
  Conn1 : PMIOPort  Side=Left
  Conn2 : PMIOPort  Port=2  Side=Right
  Conn3 : PMIOPort  Port=3  Side=Left
  connections:
  Solar Cell/LConn2 -- Conn2/RConn1
  Solar Cell/LConn1 -- Conn1/RConn1 -- Solar Cell2/LConn1 -- Solar Cell1/LConn1
  Solar Cell1/RConn1 -- Solar Cell2/LConn2
  Solar Cell/RConn1 -- Solar Cell1/LConn2
  Solar Cell2/RConn1 -- Conn3/RConn1

== system PV_solarpannel/Subsystem/Subsystem9/Subsystem5 ==
  Solar Cell : ee_lib/Sources/Solar Cell  prm=1  Isc=6 A  Voc=0.6 V  Is=1e-6 A  Is2=0 A  Iph=7.34 A  Ir0=1000 W/m^2  ec=1.5  N2=2  Rs=0 Ohm  Rp=Inf Ohm  N_series=1  TIPH1=0 1/K  EG=1.11 eV  TXIS1=3  TXIS2=3  TRS1=0  TRP1=0  Tmeas=25 C  TFIXED=25 C  thermal_mass=100 J/K  initial_temperature=25 degC
      settings: SourceProductName=Simscape Electrical  SourceProductBaseCode=PS
  Solar Cell1 : ee_lib/Sources/Solar Cell  prm=1  Isc=6 A  Voc=0.6 V  Is=1e-6 A  Is2=0 A  Iph=7.34 A  Ir0=1000 W/m^2  ec=1.5  N2=2  Rs=0 Ohm  Rp=Inf Ohm  N_series=1  TIPH1=0 1/K  EG=1.11 eV  TXIS1=3  TXIS2=3  TRS1=0  TRP1=0  Tmeas=25 C  TFIXED=25 C  thermal_mass=100 J/K  initial_temperature=25 degC
      settings: SourceProductName=Simscape Electrical  SourceProductBaseCode=PS
  Solar Cell2 : ee_lib/Sources/Solar Cell  prm=1  Isc=6 A  Voc=0.6 V  Is=1e-6 A  Is2=0 A  Iph=7.34 A  Ir0=1000 W/m^2  ec=1.5  N2=2  Rs=0 Ohm  Rp=Inf Ohm  N_series=1  TIPH1=0 1/K  EG=1.11 eV  TXIS1=3  TXIS2=3  TRS1=0  TRP1=0  Tmeas=25 C  TFIXED=25 C  thermal_mass=100 J/K  initial_temperature=25 degC
      settings: SourceProductName=Simscape Electrical  SourceProductBaseCode=PS
  Conn1 : PMIOPort  Side=Left
  Conn2 : PMIOPort  Port=2  Side=Right
  Conn3 : PMIOPort  Port=3  Side=Left
  connections:
  Solar Cell/LConn2 -- Conn2/RConn1
  Solar Cell/LConn1 -- Conn1/RConn1 -- Solar Cell2/LConn1 -- Solar Cell1/LConn1
  Solar Cell1/RConn1 -- Solar Cell2/LConn2
  Solar Cell/RConn1 -- Solar Cell1/LConn2
  Solar Cell2/RConn1 -- Conn3/RConn1

== system PV_solarpannel/Subsystem/Subsystem9/Subsystem6 ==
  Solar Cell : ee_lib/Sources/Solar Cell  prm=1  Isc=6 A  Voc=0.6 V  Is=1e-6 A  Is2=0 A  Iph=7.34 A  Ir0=1000 W/m^2  ec=1.5  N2=2  Rs=0 Ohm  Rp=Inf Ohm  N_series=1  TIPH1=0 1/K  EG=1.11 eV  TXIS1=3  TXIS2=3  TRS1=0  TRP1=0  Tmeas=25 C  TFIXED=25 C  thermal_mass=100 J/K  initial_temperature=25 degC
      settings: SourceProductName=Simscape Electrical  SourceProductBaseCode=PS
  Solar Cell1 : ee_lib/Sources/Solar Cell  prm=1  Isc=6 A  Voc=0.6 V  Is=1e-6 A  Is2=0 A  Iph=7.34 A  Ir0=1000 W/m^2  ec=1.5  N2=2  Rs=0 Ohm  Rp=Inf Ohm  N_series=1  TIPH1=0 1/K  EG=1.11 eV  TXIS1=3  TXIS2=3  TRS1=0  TRP1=0  Tmeas=25 C  TFIXED=25 C  thermal_mass=100 J/K  initial_temperature=25 degC
      settings: SourceProductName=Simscape Electrical  SourceProductBaseCode=PS
  Solar Cell2 : ee_lib/Sources/Solar Cell  prm=1  Isc=6 A  Voc=0.6 V  Is=1e-6 A  Is2=0 A  Iph=7.34 A  Ir0=1000 W/m^2  ec=1.5  N2=2  Rs=0 Ohm  Rp=Inf Ohm  N_series=1  TIPH1=0 1/K  EG=1.11 eV  TXIS1=3  TXIS2=3  TRS1=0  TRP1=0  Tmeas=25 C  TFIXED=25 C  thermal_mass=100 J/K  initial_temperature=25 degC
      settings: SourceProductName=Simscape Electrical  SourceProductBaseCode=PS
  Conn1 : PMIOPort  Side=Left
  Conn2 : PMIOPort  Port=2  Side=Right
  Conn3 : PMIOPort  Port=3  Side=Left
  connections:
  Solar Cell/LConn2 -- Conn2/RConn1
  Solar Cell/LConn1 -- Conn1/RConn1 -- Solar Cell2/LConn1 -- Solar Cell1/LConn1
  Solar Cell1/RConn1 -- Solar Cell2/LConn2
  Solar Cell/RConn1 -- Solar Cell1/LConn2
  Solar Cell2/RConn1 -- Conn3/RConn1

== system PV_solarpannel/Subsystem/Subsystem9/Subsystem7 ==
  Solar Cell : ee_lib/Sources/Solar Cell  prm=1  Isc=6 A  Voc=0.6 V  Is=1e-6 A  Is2=0 A  Iph=7.34 A  Ir0=1000 W/m^2  ec=1.5  N2=2  Rs=0 Ohm  Rp=Inf Ohm  N_series=1  TIPH1=0 1/K  EG=1.11 eV  TXIS1=3  TXIS2=3  TRS1=0  TRP1=0  Tmeas=25 C  TFIXED=25 C  thermal_mass=100 J/K  initial_temperature=25 degC
      settings: SourceProductName=Simscape Electrical  SourceProductBaseCode=PS
  Solar Cell1 : ee_lib/Sources/Solar Cell  prm=1  Isc=6 A  Voc=0.6 V  Is=1e-6 A  Is2=0 A  Iph=7.34 A  Ir0=1000 W/m^2  ec=1.5  N2=2  Rs=0 Ohm  Rp=Inf Ohm  N_series=1  TIPH1=0 1/K  EG=1.11 eV  TXIS1=3  TXIS2=3  TRS1=0  TRP1=0  Tmeas=25 C  TFIXED=25 C  thermal_mass=100 J/K  initial_temperature=25 degC
      settings: SourceProductName=Simscape Electrical  SourceProductBaseCode=PS
  Solar Cell2 : ee_lib/Sources/Solar Cell  prm=1  Isc=6 A  Voc=0.6 V  Is=1e-6 A  Is2=0 A  Iph=7.34 A  Ir0=1000 W/m^2  ec=1.5  N2=2  Rs=0 Ohm  Rp=Inf Ohm  N_series=1  TIPH1=0 1/K  EG=1.11 eV  TXIS1=3  TXIS2=3  TRS1=0  TRP1=0  Tmeas=25 C  TFIXED=25 C  thermal_mass=100 J/K  initial_temperature=25 degC
      settings: SourceProductName=Simscape Electrical  SourceProductBaseCode=PS
  Conn1 : PMIOPort  Side=Left
  Conn2 : PMIOPort  Port=2  Side=Right
  Conn3 : PMIOPort  Port=3  Side=Left
  connections:
  Solar Cell/LConn2 -- Conn2/RConn1
  Solar Cell/LConn1 -- Conn1/RConn1 -- Solar Cell2/LConn1 -- Solar Cell1/LConn1
  Solar Cell1/RConn1 -- Solar Cell2/LConn2
  Solar Cell/RConn1 -- Solar Cell1/LConn2
  Solar Cell2/RConn1 -- Conn3/RConn1

== system PV_solarpannel/Subsystem/Subsystem9/Subsystem8 ==
  Solar Cell : ee_lib/Sources/Solar Cell  prm=1  Isc=6 A  Voc=0.6 V  Is=1e-6 A  Is2=0 A  Iph=7.34 A  Ir0=1000 W/m^2  ec=1.5  N2=2  Rs=0 Ohm  Rp=Inf Ohm  N_series=1  TIPH1=0 1/K  EG=1.11 eV  TXIS1=3  TXIS2=3  TRS1=0  TRP1=0  Tmeas=25 C  TFIXED=25 C  thermal_mass=100 J/K  initial_temperature=25 degC
      settings: SourceProductName=Simscape Electrical  SourceProductBaseCode=PS
  Solar Cell1 : ee_lib/Sources/Solar Cell  prm=1  Isc=6 A  Voc=0.6 V  Is=1e-6 A  Is2=0 A  Iph=7.34 A  Ir0=1000 W/m^2  ec=1.5  N2=2  Rs=0 Ohm  Rp=Inf Ohm  N_series=1  TIPH1=0 1/K  EG=1.11 eV  TXIS1=3  TXIS2=3  TRS1=0  TRP1=0  Tmeas=25 C  TFIXED=25 C  thermal_mass=100 J/K  initial_temperature=25 degC
      settings: SourceProductName=Simscape Electrical  SourceProductBaseCode=PS
  Solar Cell2 : ee_lib/Sources/Solar Cell  prm=1  Isc=6 A  Voc=0.6 V  Is=1e-6 A  Is2=0 A  Iph=7.34 A  Ir0=1000 W/m^2  ec=1.5  N2=2  Rs=0 Ohm  Rp=Inf Ohm  N_series=1  TIPH1=0 1/K  EG=1.11 eV  TXIS1=3  TXIS2=3  TRS1=0  TRP1=0  Tmeas=25 C  TFIXED=25 C  thermal_mass=100 J/K  initial_temperature=25 degC
      settings: SourceProductName=Simscape Electrical  SourceProductBaseCode=PS
  Conn1 : PMIOPort  Side=Left
  Conn2 : PMIOPort  Port=2  Side=Right
  Conn3 : PMIOPort  Port=3  Side=Left
  connections:
  Solar Cell/LConn2 -- Conn2/RConn1
  Solar Cell/LConn1 -- Conn1/RConn1 -- Solar Cell2/LConn1 -- Solar Cell1/LConn1
  Solar Cell1/RConn1 -- Solar Cell2/LConn2
  Solar Cell/RConn1 -- Solar Cell1/LConn2
  Solar Cell2/RConn1 -- Conn3/RConn1

== system PV_solarpannel/Subsystem1/Subsystem9/Subsystem ==
  Solar Cell : ee_lib/Sources/Solar Cell  prm=1  Isc=6 A  Voc=0.6 V  Is=1e-6 A  Is2=0 A  Iph=7.34 A  Ir0=1000 W/m^2  ec=1.5  N2=2  Rs=0 Ohm  Rp=Inf Ohm  N_series=1  TIPH1=0 1/K  EG=1.11 eV  TXIS1=3  TXIS2=3  TRS1=0  TRP1=0  Tmeas=25 C  TFIXED=25 C  thermal_mass=100 J/K  initial_temperature=25 degC
      settings: SourceProductName=Simscape Electrical  SourceProductBaseCode=PS
  Solar Cell1 : ee_lib/Sources/Solar Cell  prm=1  Isc=6 A  Voc=0.6 V  Is=1e-6 A  Is2=0 A  Iph=7.34 A  Ir0=1000 W/m^2  ec=1.5  N2=2  Rs=0 Ohm  Rp=Inf Ohm  N_series=1  TIPH1=0 1/K  EG=1.11 eV  TXIS1=3  TXIS2=3  TRS1=0  TRP1=0  Tmeas=25 C  TFIXED=25 C  thermal_mass=100 J/K  initial_temperature=25 degC
      settings: SourceProductName=Simscape Electrical  SourceProductBaseCode=PS
  Solar Cell2 : ee_lib/Sources/Solar Cell  prm=1  Isc=6 A  Voc=0.6 V  Is=1e-6 A  Is2=0 A  Iph=7.34 A  Ir0=1000 W/m^2  ec=1.5  N2=2  Rs=0 Ohm  Rp=Inf Ohm  N_series=1  TIPH1=0 1/K  EG=1.11 eV  TXIS1=3  TXIS2=3  TRS1=0  TRP1=0  Tmeas=25 C  TFIXED=25 C  thermal_mass=100 J/K  initial_temperature=25 degC
      settings: SourceProductName=Simscape Electrical  SourceProductBaseCode=PS
  Conn1 : PMIOPort  Side=Left
  Conn2 : PMIOPort  Port=2  Side=Right
  Conn3 : PMIOPort  Port=3  Side=Left
  connections:
  Solar Cell/LConn2 -- Conn2/RConn1
  Solar Cell/LConn1 -- Conn1/RConn1 -- Solar Cell2/LConn1 -- Solar Cell1/LConn1
  Solar Cell1/RConn1 -- Solar Cell2/LConn2
  Solar Cell/RConn1 -- Solar Cell1/LConn2
  Solar Cell2/RConn1 -- Conn3/RConn1

== system PV_solarpannel/Subsystem1/Subsystem9/Subsystem1 ==
  Solar Cell : ee_lib/Sources/Solar Cell  prm=1  Isc=6 A  Voc=0.6 V  Is=1e-6 A  Is2=0 A  Iph=7.34 A  Ir0=1000 W/m^2  ec=1.5  N2=2  Rs=0 Ohm  Rp=Inf Ohm  N_series=1  TIPH1=0 1/K  EG=1.11 eV  TXIS1=3  TXIS2=3  TRS1=0  TRP1=0  Tmeas=25 C  TFIXED=25 C  thermal_mass=100 J/K  initial_temperature=25 degC
      settings: SourceProductName=Simscape Electrical  SourceProductBaseCode=PS
  Solar Cell1 : ee_lib/Sources/Solar Cell  prm=1  Isc=6 A  Voc=0.6 V  Is=1e-6 A  Is2=0 A  Iph=7.34 A  Ir0=1000 W/m^2  ec=1.5  N2=2  Rs=0 Ohm  Rp=Inf Ohm  N_series=1  TIPH1=0 1/K  EG=1.11 eV  TXIS1=3  TXIS2=3  TRS1=0  TRP1=0  Tmeas=25 C  TFIXED=25 C  thermal_mass=100 J/K  initial_temperature=25 degC
      settings: SourceProductName=Simscape Electrical  SourceProductBaseCode=PS
  Solar Cell2 : ee_lib/Sources/Solar Cell  prm=1  Isc=6 A  Voc=0.6 V  Is=1e-6 A  Is2=0 A  Iph=7.34 A  Ir0=1000 W/m^2  ec=1.5  N2=2  Rs=0 Ohm  Rp=Inf Ohm  N_series=1  TIPH1=0 1/K  EG=1.11 eV  TXIS1=3  TXIS2=3  TRS1=0  TRP1=0  Tmeas=25 C  TFIXED=25 C  thermal_mass=100 J/K  initial_temperature=25 degC
      settings: SourceProductName=Simscape Electrical  SourceProductBaseCode=PS
  Conn1 : PMIOPort  Side=Left
  Conn2 : PMIOPort  Port=2  Side=Right
  Conn3 : PMIOPort  Port=3  Side=Left
  connections:
  Solar Cell2/RConn1 -- Conn3/RConn1
  Solar Cell/RConn1 -- Solar Cell1/LConn2
  Solar Cell1/RConn1 -- Solar Cell2/LConn2
  Conn1/RConn1 -- Solar Cell/LConn1 -- Solar Cell1/LConn1 -- Solar Cell2/LConn1
  Solar Cell/LConn2 -- Conn2/RConn1

== system PV_solarpannel/Subsystem1/Subsystem9/Subsystem2 ==
  Solar Cell : ee_lib/Sources/Solar Cell  prm=1  Isc=6 A  Voc=0.6 V  Is=1e-6 A  Is2=0 A  Iph=7.34 A  Ir0=1000 W/m^2  ec=1.5  N2=2  Rs=0 Ohm  Rp=Inf Ohm  N_series=1  TIPH1=0 1/K  EG=1.11 eV  TXIS1=3  TXIS2=3  TRS1=0  TRP1=0  Tmeas=25 C  TFIXED=25 C  thermal_mass=100 J/K  initial_temperature=25 degC
      settings: SourceProductName=Simscape Electrical  SourceProductBaseCode=PS
  Solar Cell1 : ee_lib/Sources/Solar Cell  prm=1  Isc=6 A  Voc=0.6 V  Is=1e-6 A  Is2=0 A  Iph=7.34 A  Ir0=1000 W/m^2  ec=1.5  N2=2  Rs=0 Ohm  Rp=Inf Ohm  N_series=1  TIPH1=0 1/K  EG=1.11 eV  TXIS1=3  TXIS2=3  TRS1=0  TRP1=0  Tmeas=25 C  TFIXED=25 C  thermal_mass=100 J/K  initial_temperature=25 degC
      settings: SourceProductName=Simscape Electrical  SourceProductBaseCode=PS
  Solar Cell2 : ee_lib/Sources/Solar Cell  prm=1  Isc=6 A  Voc=0.6 V  Is=1e-6 A  Is2=0 A  Iph=7.34 A  Ir0=1000 W/m^2  ec=1.5  N2=2  Rs=0 Ohm  Rp=Inf Ohm  N_series=1  TIPH1=0 1/K  EG=1.11 eV  TXIS1=3  TXIS2=3  TRS1=0  TRP1=0  Tmeas=25 C  TFIXED=25 C  thermal_mass=100 J/K  initial_temperature=25 degC
      settings: SourceProductName=Simscape Electrical  SourceProductBaseCode=PS
  Conn1 : PMIOPort  Side=Left
  Conn2 : PMIOPort  Port=2  Side=Right
  Conn3 : PMIOPort  Port=3  Side=Left
  connections:
  Solar Cell/LConn2 -- Conn2/RConn1
  Solar Cell2/LConn1 -- Solar Cell1/LConn1 -- Solar Cell/LConn1 -- Conn1/RConn1
  Solar Cell1/RConn1 -- Solar Cell2/LConn2
  Solar Cell/RConn1 -- Solar Cell1/LConn2
  Solar Cell2/RConn1 -- Conn3/RConn1

== system PV_solarpannel/Subsystem1/Subsystem9/Subsystem3 ==
  Solar Cell : ee_lib/Sources/Solar Cell  prm=1  Isc=6 A  Voc=0.6 V  Is=1e-6 A  Is2=0 A  Iph=7.34 A  Ir0=1000 W/m^2  ec=1.5  N2=2  Rs=0 Ohm  Rp=Inf Ohm  N_series=1  TIPH1=0 1/K  EG=1.11 eV  TXIS1=3  TXIS2=3  TRS1=0  TRP1=0  Tmeas=25 C  TFIXED=25 C  thermal_mass=100 J/K  initial_temperature=25 degC
      settings: SourceProductName=Simscape Electrical  SourceProductBaseCode=PS
  Solar Cell1 : ee_lib/Sources/Solar Cell  prm=1  Isc=6 A  Voc=0.6 V  Is=1e-6 A  Is2=0 A  Iph=7.34 A  Ir0=1000 W/m^2  ec=1.5  N2=2  Rs=0 Ohm  Rp=Inf Ohm  N_series=1  TIPH1=0 1/K  EG=1.11 eV  TXIS1=3  TXIS2=3  TRS1=0  TRP1=0  Tmeas=25 C  TFIXED=25 C  thermal_mass=100 J/K  initial_temperature=25 degC
      settings: SourceProductName=Simscape Electrical  SourceProductBaseCode=PS
  Solar Cell2 : ee_lib/Sources/Solar Cell  prm=1  Isc=6 A  Voc=0.6 V  Is=1e-6 A  Is2=0 A  Iph=7.34 A  Ir0=1000 W/m^2  ec=1.5  N2=2  Rs=0 Ohm  Rp=Inf Ohm  N_series=1  TIPH1=0 1/K  EG=1.11 eV  TXIS1=3  TXIS2=3  TRS1=0  TRP1=0  Tmeas=25 C  TFIXED=25 C  thermal_mass=100 J/K  initial_temperature=25 degC
      settings: SourceProductName=Simscape Electrical  SourceProductBaseCode=PS
  Conn1 : PMIOPort  Side=Left
  Conn2 : PMIOPort  Port=2  Side=Right
  Conn3 : PMIOPort  Port=3  Side=Left
  connections:
  Solar Cell/LConn2 -- Conn2/RConn1
  Solar Cell/LConn1 -- Conn1/RConn1 -- Solar Cell2/LConn1 -- Solar Cell1/LConn1
  Solar Cell1/RConn1 -- Solar Cell2/LConn2
  Solar Cell/RConn1 -- Solar Cell1/LConn2
  Solar Cell2/RConn1 -- Conn3/RConn1
